simulink library "aerolibwindfilters"  (Simulink 6.0)
settings: Solver=ode45  SolverMode=SingleTasking  StartTime=0.0  StopTime=10.0  RelTol=1e-3
undefined symbols (not defined in the file or in its folder): dt, T_on
settings Model: Creator=sgage  LastModifiedBy=sgage  ExtModeAutoUpdateStatusClock=off
settings DataIOCC: SignalLoggingName=logsOut
settings OptimizationCC: BooleanDataType=off
settings DebuggingCC: CheckExecutionContextPreStartOutputMsg=on  CheckExecutionContextRuntimeOutputMsg=on  SolverPrmCheckMsg=none
settings HardwareCC: TargetUnknown=on
settings GRTTargetCC: LifeSpan=inf
settings SFSimCC: SFSimApplyToAllLibs=on  SFSimBuildMode=Incremental

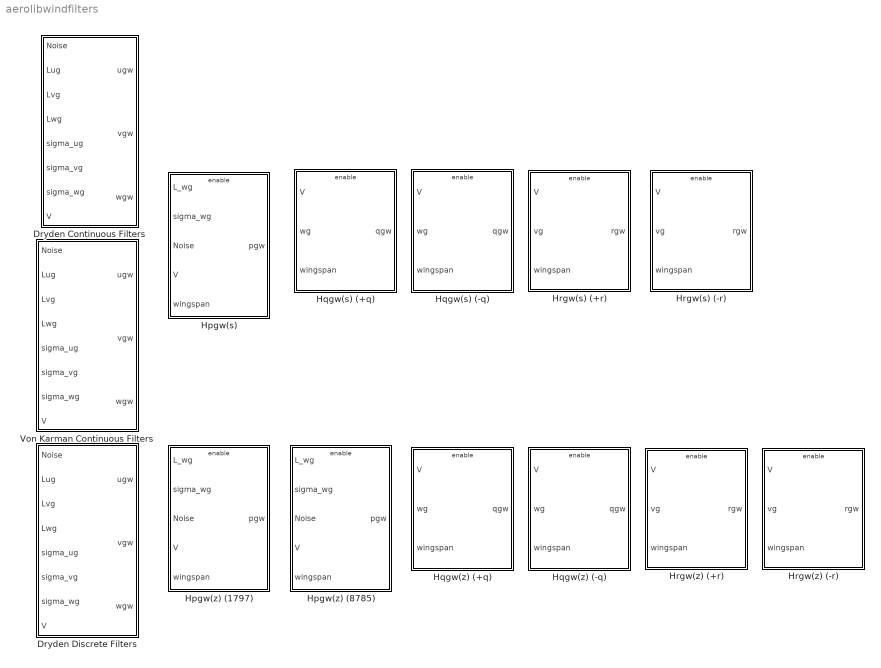
== system aerolibwindfilters ==
  Dryden Continuous Filters : Subsystem  PropExecContextAcrossSSBoundary=on
      mask Type: Dryden Continuous Filters
      mask Display: disp('Dryden\nCont.')
  Dryden Discrete Filters : Subsystem  PropExecContextAcrossSSBoundary=on
      mask Type: Dryden Discrete Filters
      mask Display: disp('Dryden\nDiscrete')
  Hpgw(s) : Subsystem  PropExecContextAcrossSSBoundary=on
      mask Type: Hpgw(s)
      mask Display: disp('P Cont.')
  Hpgw(z) (1797) : Subsystem  PropExecContextAcrossSSBoundary=on
      mask Type: Hpqw(z)
      mask Display: disp('P Disc.\n(1797)')
  Hpgw(z) (8785) : Subsystem  PropExecContextAcrossSSBoundary=on
      mask Type: Hpqw(z)
      mask Display: disp('P Disc.\n(8785)')
  Hqgw(s) (+q) : Subsystem  PropExecContextAcrossSSBoundary=on
      mask Type: Hqgw(s) (+q)
      mask Display: disp('+Q Cont.')
  Hqgw(s) (-q) : Subsystem  PropExecContextAcrossSSBoundary=on
      mask Type: Hqgw(s) (-q)
      mask Display: disp('-Q Cont.')
  Hqgw(z) (+q) : Subsystem  PropExecContextAcrossSSBoundary=on
      mask Type: Hqgw(z) (+q)
      mask Display: disp('+Q Disc.')
  Hqgw(z) (-q) : Subsystem  PropExecContextAcrossSSBoundary=on
      mask Type: Hqgw(z) (-q)
      mask Display: disp('-Q Disc.')
  Hrgw(s) (+r) : Subsystem  PropExecContextAcrossSSBoundary=on
      mask Type: Hrgw(s) (+r)
      mask Display: disp('+R Cont.')
  Hrgw(s) (-r) : Subsystem  PropExecContextAcrossSSBoundary=on
      mask Type: Hrgw(s) (-r)
      mask Display: disp('-R Cont.')
  Hrgw(z) (+r) : Subsystem  PropExecContextAcrossSSBoundary=on
      mask Type: Hrgw(z) (+r)
      mask Display: disp('+R Disc.')
  Hrgw(z) (-r) : Subsystem  PropExecContextAcrossSSBoundary=on
      mask Type: Hrgw(z) (-r)
      mask Display: disp('-R Disc.')
  Von Karman Continuous Filters : Subsystem  PropExecContextAcrossSSBoundary=on
      mask Type: Von Karman Continuous Filters
      mask Display: disp('VonKarman\nCont.')

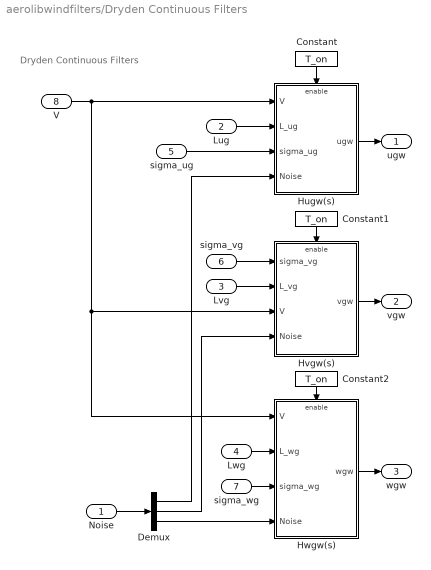
== system aerolibwindfilters/Dryden Continuous Filters ==
  note: Dryden Continuous Filters
  Noise : Inport  LatchInput=off
  Lug : Inport  Port=2  LatchInput=off
  Lvg : Inport  Port=3  LatchInput=off
  Lwg : Inport  Port=4  LatchInput=off
  sigma_ug : Inport  Port=5  LatchInput=off
  sigma_vg : Inport  Port=6  LatchInput=off
  sigma_wg : Inport  Port=7  LatchInput=off
  V : Inport  Port=8  LatchInput=off
  Constant : Constant  Orientation=down  Value=T_on
  Constant1 : Constant  Orientation=down  Value=T_on
  Constant2 : Constant  Orientation=down  Value=T_on
  Demux : Demux  Outputs=3
  Hugw(s) : Subsystem  PropExecContextAcrossSSBoundary=on
  Hvgw(s) : Subsystem  PropExecContextAcrossSSBoundary=on
  Hwgw(s) : Subsystem  PropExecContextAcrossSSBoundary=on
  ugw : Outport  OutputWhenDisabled=reset  InitialOutput=0
  vgw : Outport  Port=2  OutputWhenDisabled=reset  InitialOutput=0
  wgw : Outport  Port=3  OutputWhenDisabled=reset  InitialOutput=0
  wires:
  sigma_wg/1 -> Hwgw(s)/3(sigma_wg)
  Lwg/1 -> Hwgw(s)/2(L_wg)
  sigma_ug/1 -> Hugw(s)/3(sigma_ug)
  Lug/1 -> Hugw(s)/2(L_ug)
  V/1 -> Hwgw(s)/1(V), Hvgw(s)/3(V), Hugw(s)/1(V)
  Demux/3 -> Hwgw(s)/4(Noise)
  Hugw(s)/1(ugw) -> ugw/1
  Hvgw(s)/1(vgw) -> vgw/1
  Hwgw(s)/1(wgw) -> wgw/1
  Noise/1 -> Demux/1
  Demux/1 -> Hugw(s)/4(Noise)
  Demux/2 -> Hvgw(s)/4(Noise)
  Constant/1 -> Hugw(s)/Enable
  Constant1/1 -> Hvgw(s)/Enable
  Constant2/1 -> Hwgw(s)/Enable
  Lvg/1 -> Hvgw(s)/2(L_vg)
  sigma_vg/1 -> Hvgw(s)/1(sigma_vg)

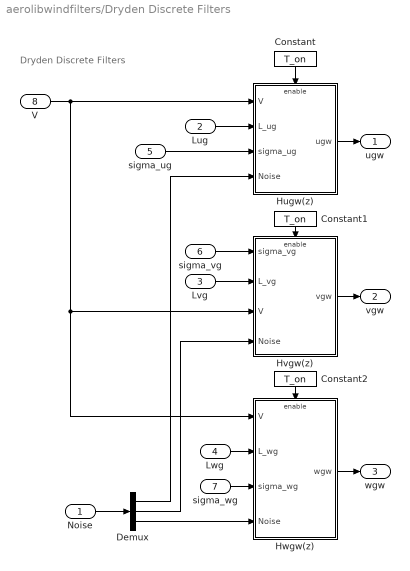
== system aerolibwindfilters/Dryden Discrete Filters ==
  note: Dryden Discrete Filters
  Noise : Inport  LatchInput=off
  Lug : Inport  Port=2  LatchInput=off
  Lvg : Inport  Port=3  LatchInput=off
  Lwg : Inport  Port=4  LatchInput=off
  sigma_ug : Inport  Port=5  LatchInput=off
  sigma_vg : Inport  Port=6  LatchInput=off
  sigma_wg : Inport  Port=7  LatchInput=off
  V : Inport  Port=8  LatchInput=off
  Constant : Constant  Orientation=down  Value=T_on
  Constant1 : Constant  Orientation=down  Value=T_on
  Constant2 : Constant  Orientation=down  Value=T_on
  Demux : Demux  Outputs=3
  Hugw(z) : Subsystem  PropExecContextAcrossSSBoundary=on
  Hvgw(z) : Subsystem  PropExecContextAcrossSSBoundary=on
  Hwgw(z) : Subsystem  PropExecContextAcrossSSBoundary=on
  ugw : Outport  InitialOutput=0
  vgw : Outport  Port=2  InitialOutput=0
  wgw : Outport  Port=3  InitialOutput=0
  wires:
  Lvg/1 -> Hvgw(z)/2(L_vg)
  Constant2/1 -> Hwgw(z)/Enable
  Constant1/1 -> Hvgw(z)/Enable
  Constant/1 -> Hugw(z)/Enable
  Demux/2 -> Hvgw(z)/4(Noise)
  Demux/1 -> Hugw(z)/4(Noise)
  Noise/1 -> Demux/1
  Hwgw(z)/1(wgw) -> wgw/1
  Hvgw(z)/1(vgw) -> vgw/1
  Hugw(z)/1(ugw) -> ugw/1
  Demux/3 -> Hwgw(z)/4(Noise)
  V/1 -> Hugw(z)/1(V), Hwgw(z)/1(V), Hvgw(z)/3(V)
  Lug/1 -> Hugw(z)/2(L_ug)
  sigma_ug/1 -> Hugw(z)/3(sigma_ug)
  Lwg/1 -> Hwgw(z)/2(L_wg)
  sigma_wg/1 -> Hwgw(z)/3(sigma_wg)
  sigma_vg/1 -> Hvgw(z)/1(sigma_vg)

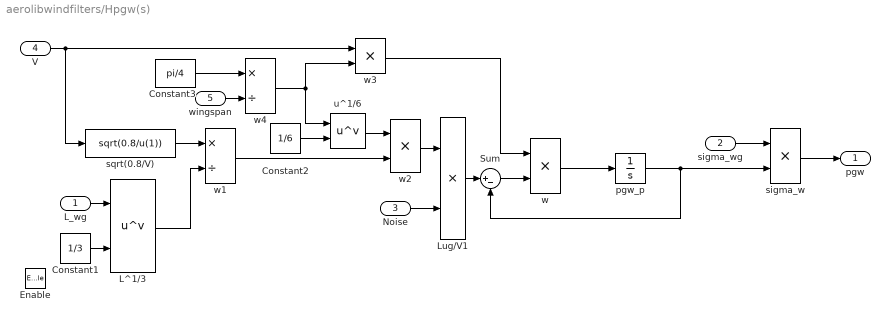
== system aerolibwindfilters/Hpgw(s) ==
  L_wg : Inport  LatchInput=off
  sigma_wg : Inport  Port=2  LatchInput=off
  Noise : Inport  Port=3  LatchInput=off
  V : Inport  Port=4  LatchInput=off
  wingspan : Inport  Port=5  LatchInput=off
  Enable : EnablePort  StatesWhenEnabling=reset
  Constant1 : Constant  Value=1/3
  Constant2 : Constant  Value=1/6
  Constant3 : Constant  Value=pi/4
  L^1/3 : Math  Operator=pow  SaturateOnIntegerOverflow=on
  Lug/V1 : Product  SaturateOnIntegerOverflow=on  InputSameDT=on
  Sum : Sum  Inputs=|+-  SaturateOnIntegerOverflow=on  InputSameDT=on
  pgw_p : Integrator
  sigma_w : Product  SaturateOnIntegerOverflow=on  InputSameDT=on
  sqrt(0.8/V) : Fcn  Expr=sqrt(0.8/u(1))
  u^1/6 : Math  Operator=pow  SaturateOnIntegerOverflow=on
  w : Product  SaturateOnIntegerOverflow=on  InputSameDT=on
  w1 : Product  Inputs=*/  SaturateOnIntegerOverflow=on  InputSameDT=on
  w2 : Product  SaturateOnIntegerOverflow=on  InputSameDT=on
  w3 : Product  SaturateOnIntegerOverflow=on  InputSameDT=on
  w4 : Product  Inputs=*/  SaturateOnIntegerOverflow=on  InputSameDT=on
  pgw : Outport  OutputWhenDisabled=reset  InitialOutput=0
  wires:
  wingspan/1 -> w4/2
  L^1/3/1 -> w1/2
  Noise/1 -> Lug/V1/2
  sqrt(0.8/V)/1 -> w1/1
  L_wg/1 -> L^1/3/1
  sigma_wg/1 -> sigma_w/1
  sigma_w/1 -> pgw/1
  w3/1 -> w/1
  Constant1/1 -> L^1/3/2
  pgw_p/1 -> Sum/2, sigma_w/2
  V/1 -> sqrt(0.8/V)/1, w3/1
  w/1 -> pgw_p/1
  Lug/V1/1 -> Sum/1
  Sum/1 -> w/2
  Constant2/1 -> u^1/6/2
  Constant3/1 -> w4/1
  w4/1 -> w3/2, u^1/6/1
  w2/1 -> Lug/V1/1
  u^1/6/1 -> w2/1
  w1/1 -> w2/2

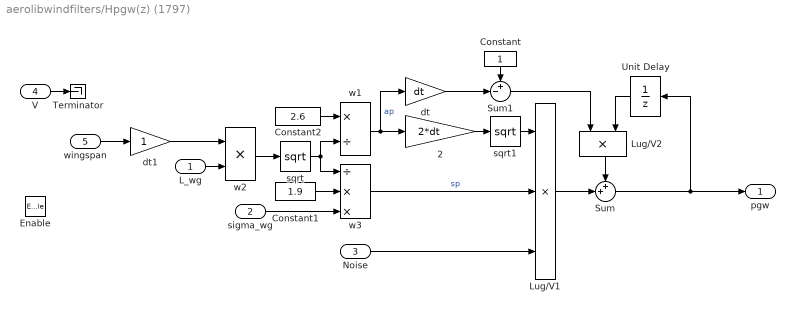
== system aerolibwindfilters/Hpgw(z) (1797) ==
  L_wg : Inport  LatchInput=off
  sigma_wg : Inport  Port=2  LatchInput=off
  Noise : Inport  Port=3  LatchInput=off
  V : Inport  Port=4  LatchInput=off
  wingspan : Inport  Port=5  LatchInput=off
  Enable : EnablePort  StatesWhenEnabling=reset
  2 : Gain  Gain=2*dt  SaturateOnIntegerOverflow=on
  Constant : Constant  Orientation=down
  Constant1 : Constant  Value=1.9
  Constant2 : Constant  Value=2.6
  Lug/V1 : Product  Inputs=3  SaturateOnIntegerOverflow=on  InputSameDT=on
  Lug/V2 : Product  Orientation=down  SaturateOnIntegerOverflow=on  InputSameDT=on
  Sum : Sum  Inputs=++|  SaturateOnIntegerOverflow=on  InputSameDT=on
  Sum1 : Sum  Inputs=+-|  SaturateOnIntegerOverflow=on  InputSameDT=on
  Terminator : Terminator
  Unit Delay : UnitDelay  Orientation=left  SampleTime=dt
  dt : Gain  Gain=dt  SaturateOnIntegerOverflow=on
  dt1 : Gain  SaturateOnIntegerOverflow=on
  sqrt : Math  Operator=sqrt  SaturateOnIntegerOverflow=on
  sqrt1 : Math  Operator=sqrt  SaturateOnIntegerOverflow=on
  w1 : Product  Inputs=*/  SaturateOnIntegerOverflow=on  InputSameDT=on
  w2 : Product  SaturateOnIntegerOverflow=on  InputSameDT=on
  w3 : Product  Inputs=/**  SaturateOnIntegerOverflow=on  InputSameDT=on
  pgw : Outport  OutputWhenDisabled=reset  InitialOutput=0
  wires:
  wingspan/1 -> dt1/1
  Lug/V2/1 -> Sum/1
  Unit Delay/1 -> Lug/V2/2
  Constant/1 -> Sum1/1
  Sum1/1 -> Lug/V2/1
  2/1 -> sqrt1/1
  dt/1 -> Sum1/2
  sqrt1/1 -> Lug/V1/1
  sigma_wg/1 -> w3/3
  w3/1 -> Lug/V1/2  "sp"
  Constant1/1 -> w3/2
  w1/1 -> 2/1, dt/1  "ap"
  Constant2/1 -> w1/1
  sqrt/1 -> w3/1, w1/2
  w2/1 -> sqrt/1
  L_wg/1 -> w2/2
  V/1 -> Terminator/1
  dt1/1 -> w2/1
  Lug/V1/1 -> Sum/2
  Sum/1 -> Unit Delay/1, pgw/1
  Noise/1 -> Lug/V1/3

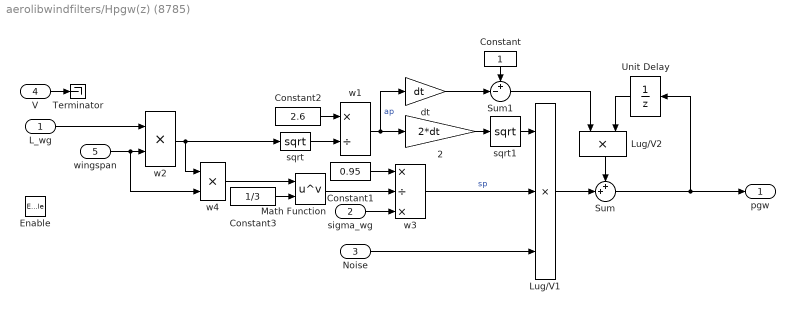
== system aerolibwindfilters/Hpgw(z) (8785) ==
  L_wg : Inport  LatchInput=off
  sigma_wg : Inport  Port=2  LatchInput=off
  Noise : Inport  Port=3  LatchInput=off
  V : Inport  Port=4  LatchInput=off
  wingspan : Inport  Port=5  LatchInput=off
  Enable : EnablePort  StatesWhenEnabling=reset
  2 : Gain  Gain=2*dt  SaturateOnIntegerOverflow=on
  Constant : Constant  Orientation=down
  Constant1 : Constant  Value=0.95
  Constant2 : Constant  Value=2.6
  Constant3 : Constant  Value=1/3
  Lug/V1 : Product  Inputs=3  SaturateOnIntegerOverflow=on  InputSameDT=on
  Lug/V2 : Product  Orientation=down  SaturateOnIntegerOverflow=on  InputSameDT=on
  Math Function : Math  Operator=pow  SaturateOnIntegerOverflow=on
  Sum : Sum  Inputs=++|  SaturateOnIntegerOverflow=on  InputSameDT=on
  Sum1 : Sum  Inputs=+-|  SaturateOnIntegerOverflow=on  InputSameDT=on
  Terminator : Terminator
  Unit Delay : UnitDelay  Orientation=left  SampleTime=dt
  dt : Gain  Gain=dt  SaturateOnIntegerOverflow=on
  sqrt : Math  Operator=sqrt  SaturateOnIntegerOverflow=on
  sqrt1 : Math  Operator=sqrt  SaturateOnIntegerOverflow=on
  w1 : Product  Inputs=*/  SaturateOnIntegerOverflow=on  InputSameDT=on
  w2 : Product  SaturateOnIntegerOverflow=on  InputSameDT=on
  w3 : Product  Inputs=*/*  SaturateOnIntegerOverflow=on  InputSameDT=on
  w4 : Product  SaturateOnIntegerOverflow=on  InputSameDT=on
  pgw : Outport  OutputWhenDisabled=reset  InitialOutput=0
  wires:
  Noise/1 -> Lug/V1/3
  Sum/1 -> pgw/1, Unit Delay/1
  Lug/V1/1 -> Sum/2
  V/1 -> Terminator/1
  wingspan/1 -> w2/2, w4/2
  w2/1 -> sqrt/1, w4/1
  sqrt/1 -> w1/2
  Constant2/1 -> w1/1
  w1/1 -> dt/1, 2/1  "ap"
  Constant1/1 -> w3/1
  w3/1 -> Lug/V1/2  "sp"
  sigma_wg/1 -> w3/3
  sqrt1/1 -> Lug/V1/1
  dt/1 -> Sum1/2
  2/1 -> sqrt1/1
  Sum1/1 -> Lug/V2/1
  Constant/1 -> Sum1/1
  Unit Delay/1 -> Lug/V2/2
  Lug/V2/1 -> Sum/1
  L_wg/1 -> w2/1
  Math Function/1 -> w3/2
  w4/1 -> Math Function/1
  Constant3/1 -> Math Function/2

== system aerolibwindfilters/Hqgw(s) (+q) ==
  V : Inport  LatchInput=off
  wg : Inport  Port=2  LatchInput=off
  wingspan : Inport  Port=3  LatchInput=off
  Enable : EnablePort  StatesWhenEnabling=reset
  Sum : Sum  Inputs=|+-  SaturateOnIntegerOverflow=on  InputSameDT=on
  pi/4 : Gain  Gain=pi/4  SaturateOnIntegerOverflow=on
  qgw_p : Integrator
  w : Product  Inputs=/**  SaturateOnIntegerOverflow=on  InputSameDT=on
  wg/V : Product  Inputs=/*  SaturateOnIntegerOverflow=on  InputSameDT=on
  qgw : Outport  OutputWhenDisabled=reset  InitialOutput=0
  wires:
  wingspan/1 -> w/1
  wg/1 -> wg/V/2
  wg/V/1 -> Sum/1
  Sum/1 -> w/3
  w/1 -> qgw/1, qgw_p/1
  V/1 -> wg/V/1, pi/4/1
  qgw_p/1 -> Sum/2
  pi/4/1 -> w/2

== system aerolibwindfilters/Hqgw(s) (-q) ==
  V : Inport  LatchInput=off
  wg : Inport  Port=2  LatchInput=off
  wingspan : Inport  Port=3  LatchInput=off
  Enable : EnablePort  StatesWhenEnabling=reset
  -1 : Gain  Gain=-1  SaturateOnIntegerOverflow=on
  Sum : Sum  Inputs=|+-  SaturateOnIntegerOverflow=on  InputSameDT=on
  pi/4 : Gain  Gain=pi/4  SaturateOnIntegerOverflow=on
  qgw_p : Integrator
  w : Product  Inputs=/**  SaturateOnIntegerOverflow=on  InputSameDT=on
  wg/V : Product  Inputs=/*  SaturateOnIntegerOverflow=on  InputSameDT=on
  qgw : Outport  OutputWhenDisabled=reset  InitialOutput=0
  wires:
  pi/4/1 -> w/2
  qgw_p/1 -> Sum/2
  V/1 -> pi/4/1, wg/V/1
  w/1 -> -1/1, qgw_p/1
  Sum/1 -> w/3
  wg/V/1 -> Sum/1
  wg/1 -> wg/V/2
  wingspan/1 -> w/1
  -1/1 -> qgw/1

== system aerolibwindfilters/Hqgw(z) (+q) ==
  V : Inport  LatchInput=off
  wg : Inport  Port=2  LatchInput=off
  wingspan : Inport  Port=3  LatchInput=off
  Enable : EnablePort  StatesWhenEnabling=reset
  Constant : Constant  Orientation=down
  Lug/V2 : Product  Orientation=down  SaturateOnIntegerOverflow=on  InputSameDT=on
  Sum1 : Sum  Inputs=++|  SaturateOnIntegerOverflow=on  InputSameDT=on
  Sum2 : Sum  Inputs=+-|  SaturateOnIntegerOverflow=on  InputSameDT=on
  Sum3 : Sum  Inputs=|+-  SaturateOnIntegerOverflow=on  InputSameDT=on
  Unit Delay : UnitDelay  Orientation=left  SampleTime=dt
  Unit Delay1 : UnitDelay  SampleTime=dt
  dt : Gain  Gain=dt  SaturateOnIntegerOverflow=on
  dt1 : Gain  Gain=4/pi  SaturateOnIntegerOverflow=on
  w1 : Product  Inputs=*/  SaturateOnIntegerOverflow=on  InputSameDT=on
  w2 : Product  Inputs=/*  SaturateOnIntegerOverflow=on  InputSameDT=on
  qgw : Outport  OutputWhenDisabled=reset  InitialOutput=0
  wires:
  wingspan/1 -> dt1/1
  wg/1 -> Unit Delay1/1, Sum3/1
  Unit Delay1/1 -> Sum3/2
  Sum3/1 -> w2/2
  w1/1 -> dt/1  "aq"
  Lug/V2/1 -> Sum1/1
  Unit Delay/1 -> Lug/V2/2
  Constant/1 -> Sum2/1
  Sum2/1 -> Lug/V2/1
  dt/1 -> Sum2/2
  w2/1 -> Sum1/2
  Sum1/1 -> qgw/1, Unit Delay/1
  dt1/1 -> w2/1, w1/2
  V/1 -> w1/1

== system aerolibwindfilters/Hqgw(z) (-q) ==
  V : Inport  LatchInput=off
  wg : Inport  Port=2  LatchInput=off
  wingspan : Inport  Port=3  LatchInput=off
  Enable : EnablePort  StatesWhenEnabling=reset
  Constant : Constant  Orientation=down
  Lug/V2 : Product  Orientation=down  SaturateOnIntegerOverflow=on  InputSameDT=on
  Sum1 : Sum  Inputs=+-|  SaturateOnIntegerOverflow=on  InputSameDT=on
  Sum2 : Sum  Inputs=+-|  SaturateOnIntegerOverflow=on  InputSameDT=on
  Sum3 : Sum  Inputs=|+-  SaturateOnIntegerOverflow=on  InputSameDT=on
  Unit Delay : UnitDelay  Orientation=left  SampleTime=dt
  Unit Delay1 : UnitDelay  SampleTime=dt
  dt : Gain  Gain=dt  SaturateOnIntegerOverflow=on
  dt1 : Gain  Gain=4/pi  SaturateOnIntegerOverflow=on
  w1 : Product  Inputs=*/  SaturateOnIntegerOverflow=on  InputSameDT=on
  w2 : Product  Inputs=/*  SaturateOnIntegerOverflow=on  InputSameDT=on
  qgw : Outport  OutputWhenDisabled=reset  InitialOutput=0
  wires:
  V/1 -> w1/1
  dt1/1 -> w1/2, w2/1
  Sum1/1 -> Unit Delay/1, qgw/1
  w2/1 -> Sum1/2
  dt/1 -> Sum2/2
  Sum2/1 -> Lug/V2/1
  Constant/1 -> Sum2/1
  Unit Delay/1 -> Lug/V2/2
  Lug/V2/1 -> Sum1/1
  w1/1 -> dt/1  "aq"
  Sum3/1 -> w2/2
  Unit Delay1/1 -> Sum3/2
  wg/1 -> Sum3/1, Unit Delay1/1
  wingspan/1 -> dt1/1

== system aerolibwindfilters/Hrgw(s) (+r) ==
  V : Inport  LatchInput=off
  vg : Inport  Port=2  LatchInput=off
  wingspan : Inport  Port=3  LatchInput=off
  Enable : EnablePort  StatesWhenEnabling=reset
  Sum : Sum  Inputs=|+-  SaturateOnIntegerOverflow=on  InputSameDT=on
  pi/3 : Gain  Gain=pi/3  SaturateOnIntegerOverflow=on
  rgw_p : Integrator
  vg/V : Product  Inputs=/*  SaturateOnIntegerOverflow=on  InputSameDT=on
  w : Product  Inputs=/**  SaturateOnIntegerOverflow=on  InputSameDT=on
  rgw : Outport  OutputWhenDisabled=reset  InitialOutput=0
  wires:
  wingspan/1 -> w/1
  vg/V/1 -> Sum/1
  vg/1 -> vg/V/2
  pi/3/1 -> w/2
  V/1 -> vg/V/1, pi/3/1
  w/1 -> rgw/1, rgw_p/1
  Sum/1 -> w/3
  rgw_p/1 -> Sum/2

== system aerolibwindfilters/Hrgw(s) (-r) ==
  V : Inport  LatchInput=off
  vg : Inport  Port=2  LatchInput=off
  wingspan : Inport  Port=3  LatchInput=off
  Enable : EnablePort  StatesWhenEnabling=reset
  -1 : Gain  Gain=-1  SaturateOnIntegerOverflow=on
  Sum : Sum  Inputs=|+-  SaturateOnIntegerOverflow=on  InputSameDT=on
  pi/3 : Gain  Gain=pi/3  SaturateOnIntegerOverflow=on
  rgw_p : Integrator
  vg/V : Product  Inputs=/*  SaturateOnIntegerOverflow=on  InputSameDT=on
  w : Product  Inputs=/**  SaturateOnIntegerOverflow=on  InputSameDT=on
  rgw : Outport  OutputWhenDisabled=reset  InitialOutput=0
  wires:
  Sum/1 -> w/3
  w/1 -> -1/1, rgw_p/1
  V/1 -> pi/3/1, vg/V/1
  rgw_p/1 -> Sum/2
  pi/3/1 -> w/2
  vg/1 -> vg/V/2
  vg/V/1 -> Sum/1
  -1/1 -> rgw/1
  wingspan/1 -> w/1

== system aerolibwindfilters/Hrgw(z) (+r) ==
  V : Inport  LatchInput=off
  vg : Inport  Port=2  LatchInput=off
  wingspan : Inport  Port=3  LatchInput=off
  Enable : EnablePort  StatesWhenEnabling=reset
  Constant : Constant  Orientation=down
  Lug/V2 : Product  Orientation=down  SaturateOnIntegerOverflow=on  InputSameDT=on
  Sum1 : Sum  Inputs=++|  SaturateOnIntegerOverflow=on  InputSameDT=on
  Sum2 : Sum  Inputs=+-|  SaturateOnIntegerOverflow=on  InputSameDT=on
  Sum3 : Sum  Inputs=|+-  SaturateOnIntegerOverflow=on  InputSameDT=on
  Unit Delay : UnitDelay  Orientation=left  SampleTime=dt
  Unit Delay1 : UnitDelay  SampleTime=dt
  dt : Gain  Gain=dt  SaturateOnIntegerOverflow=on
  dt1 : Gain  Gain=3/pi  SaturateOnIntegerOverflow=on
  w1 : Product  Inputs=*/  SaturateOnIntegerOverflow=on  InputSameDT=on
  w2 : Product  Inputs=/*  SaturateOnIntegerOverflow=on  InputSameDT=on
  rgw : Outport  OutputWhenDisabled=reset  InitialOutput=0
  wires:
  wingspan/1 -> dt1/1
  Unit Delay1/1 -> Sum3/2
  vg/1 -> Sum3/1, Unit Delay1/1
  Sum3/1 -> w2/2
  w1/1 -> dt/1  "ar"
  Lug/V2/1 -> Sum1/1
  Unit Delay/1 -> Lug/V2/2
  Constant/1 -> Sum2/1
  Sum2/1 -> Lug/V2/1
  dt/1 -> Sum2/2
  w2/1 -> Sum1/2
  Sum1/1 -> rgw/1, Unit Delay/1
  dt1/1 -> w1/2, w2/1
  V/1 -> w1/1

== system aerolibwindfilters/Hrgw(z) (-r) ==
  V : Inport  LatchInput=off
  vg : Inport  Port=2  LatchInput=off
  wingspan : Inport  Port=3  LatchInput=off
  Enable : EnablePort  StatesWhenEnabling=reset
  Constant : Constant  Orientation=down
  Lug/V2 : Product  Orientation=down  SaturateOnIntegerOverflow=on  InputSameDT=on
  Sum1 : Sum  Inputs=+-|  SaturateOnIntegerOverflow=on  InputSameDT=on
  Sum2 : Sum  Inputs=+-|  SaturateOnIntegerOverflow=on  InputSameDT=on
  Sum3 : Sum  Inputs=|+-  SaturateOnIntegerOverflow=on  InputSameDT=on
  Unit Delay : UnitDelay  Orientation=left  SampleTime=dt
  Unit Delay1 : UnitDelay  SampleTime=dt
  dt : Gain  Gain=dt  SaturateOnIntegerOverflow=on
  dt1 : Gain  Gain=3/pi  SaturateOnIntegerOverflow=on
  w1 : Product  Inputs=*/  SaturateOnIntegerOverflow=on  InputSameDT=on
  w2 : Product  Inputs=/*  SaturateOnIntegerOverflow=on  InputSameDT=on
  rgw : Outport  OutputWhenDisabled=reset  InitialOutput=0
  wires:
  wingspan/1 -> dt1/1
  V/1 -> w1/1
  dt1/1 -> w2/1, w1/2
  Sum1/1 -> Unit Delay/1, rgw/1
  w2/1 -> Sum1/2
  dt/1 -> Sum2/2
  Sum2/1 -> Lug/V2/1
  Constant/1 -> Sum2/1
  Unit Delay/1 -> Lug/V2/2
  Lug/V2/1 -> Sum1/1
  w1/1 -> dt/1  "ar"
  Sum3/1 -> w2/2
  vg/1 -> Unit Delay1/1, Sum3/1
  Unit Delay1/1 -> Sum3/2

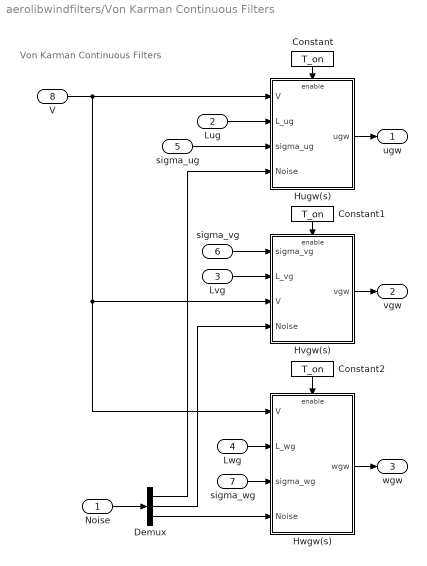
== system aerolibwindfilters/Von Karman Continuous Filters ==
  note: Von Karman Continuous Filters
  Noise : Inport  LatchInput=off
  Lug : Inport  Port=2  LatchInput=off
  Lvg : Inport  Port=3  LatchInput=off
  Lwg : Inport  Port=4  LatchInput=off
  sigma_ug : Inport  Port=5  LatchInput=off
  sigma_vg : Inport  Port=6  LatchInput=off
  sigma_wg : Inport  Port=7  LatchInput=off
  V : Inport  Port=8  LatchInput=off
  Constant : Constant  Orientation=down  Value=T_on
  Constant1 : Constant  Orientation=down  Value=T_on
  Constant2 : Constant  Orientation=down  Value=T_on
  Demux : Demux  Outputs=3
  Hugw(s) : Subsystem  PropExecContextAcrossSSBoundary=on
  Hvgw(s) : Subsystem  PropExecContextAcrossSSBoundary=on
  Hwgw(s) : Subsystem  PropExecContextAcrossSSBoundary=on
  ugw : Outport  OutputWhenDisabled=reset  InitialOutput=0
  vgw : Outport  Port=2  OutputWhenDisabled=reset  InitialOutput=0
  wgw : Outport  Port=3  OutputWhenDisabled=reset  InitialOutput=0
  wires:
  sigma_wg/1 -> Hwgw(s)/3(sigma_wg)
  Lwg/1 -> Hwgw(s)/2(L_wg)
  sigma_ug/1 -> Hugw(s)/3(sigma_ug)
  Lug/1 -> Hugw(s)/2(L_ug)
  V/1 -> Hwgw(s)/1(V), Hvgw(s)/3(V), Hugw(s)/1(V)
  Demux/3 -> Hwgw(s)/4(Noise)
  Hugw(s)/1(ugw) -> ugw/1
  Hvgw(s)/1(vgw) -> vgw/1
  Hwgw(s)/1(wgw) -> wgw/1
  Noise/1 -> Demux/1
  Demux/1 -> Hugw(s)/4(Noise)
  Demux/2 -> Hvgw(s)/4(Noise)
  Constant/1 -> Hugw(s)/Enable
  Constant2/1 -> Hwgw(s)/Enable
  Constant1/1 -> Hvgw(s)/Enable
  Lvg/1 -> Hvgw(s)/2(L_vg)
  sigma_vg/1 -> Hvgw(s)/1(sigma_vg)

== system aerolibwindfilters/Dryden Continuous Filters/Hugw(s) ==
  V : Inport  LatchInput=off
  L_ug : Inport  Port=2  LatchInput=off
  sigma_ug : Inport  Port=3  LatchInput=off
  Noise : Inport  Port=4  LatchInput=off
  Enable : EnablePort  StatesWhenEnabling=reset
  (2/pi) : Gain  Gain=2/pi  SaturateOnIntegerOverflow=on
  Lug/V : Product  Inputs=*/  SaturateOnIntegerOverflow=on  InputSameDT=on
  Lug/V1 : Product  SaturateOnIntegerOverflow=on  InputSameDT=on
  Math Function : Math  Operator=sqrt  SaturateOnIntegerOverflow=on
  Sum : Sum  Inputs=|+-  SaturateOnIntegerOverflow=on  InputSameDT=on
  ug_p : Integrator
  w : Product  Inputs=/*  SaturateOnIntegerOverflow=on  InputSameDT=on
  w1 : Product  SaturateOnIntegerOverflow=on  InputSameDT=on
  ugw : Outport  OutputWhenDisabled=reset  InitialOutput=0
  wires:
  Lug/V/1 -> w/1, (2/pi)/1
  Sum/1 -> w/2
  Lug/V1/1 -> Sum/1
  w/1 -> ug_p/1
  V/1 -> Lug/V/2
  L_ug/1 -> Lug/V/1
  ug_p/1 -> Sum/2, w1/2
  w1/1 -> ugw/1
  sigma_ug/1 -> w1/1
  Noise/1 -> Lug/V1/2
  (2/pi)/1 -> Math Function/1
  Math Function/1 -> Lug/V1/1

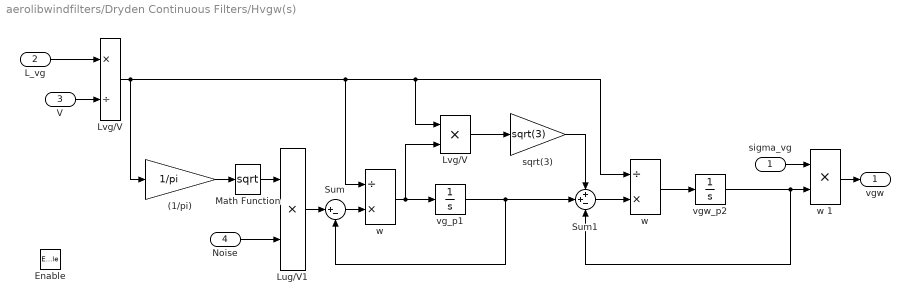
== system aerolibwindfilters/Dryden Continuous Filters/Hvgw(s) ==
  sigma_vg : Inport  LatchInput=off
  L_vg : Inport  Port=2  LatchInput=off
  V : Inport  Port=3  LatchInput=off
  Noise : Inport  Port=4  LatchInput=off
  Enable : EnablePort  StatesWhenEnabling=reset
  (1/pi) : Gain  Gain=1/pi  SaturateOnIntegerOverflow=on
  Lug/V1 : Product  SaturateOnIntegerOverflow=on  InputSameDT=on
  Lvg/V : Product  Inputs=*/  SaturateOnIntegerOverflow=on  InputSameDT=on
  "Lvg/V " : Product  SaturateOnIntegerOverflow=on  InputSameDT=on
  Math Function : Math  Operator=sqrt  SaturateOnIntegerOverflow=on
  Sum : Sum  Inputs=|+-  SaturateOnIntegerOverflow=on  InputSameDT=on
  Sum1 : Sum  Inputs=++-  SaturateOnIntegerOverflow=on  InputSameDT=on
  sqrt(3) : Gain  Gain=sqrt(3)  SaturateOnIntegerOverflow=on
  vg_p1 : Integrator
  vgw_p2 : Integrator
  w : Product  Inputs=/*  SaturateOnIntegerOverflow=on  InputSameDT=on
  "w " : Product  Inputs=/*  SaturateOnIntegerOverflow=on  InputSameDT=on
  w 1 : Product  SaturateOnIntegerOverflow=on  InputSameDT=on
  vgw : Outport  OutputWhenDisabled=reset  InitialOutput=0
  wires:
  (1/pi)/1 -> Math Function/1
  sqrt(3)/1 -> Sum1/1
  "Lvg/V "/1 -> sqrt(3)/1
  "w "/1 -> vgw_p2/1
  Sum1/1 -> "w "/2
  vgw_p2/1 -> Sum1/3, w 1/2
  vg_p1/1 -> Sum1/2, Sum/2
  L_vg/1 -> Lvg/V/1
  V/1 -> Lvg/V/2
  w/1 -> "Lvg/V "/2, vg_p1/1
  Lug/V1/1 -> Sum/1
  Sum/1 -> w/2
  Lvg/V/1 -> "Lvg/V "/1, "w "/1, w/1, (1/pi)/1
  sigma_vg/1 -> w 1/1
  Noise/1 -> Lug/V1/2
  w 1/1 -> vgw/1
  Math Function/1 -> Lug/V1/1

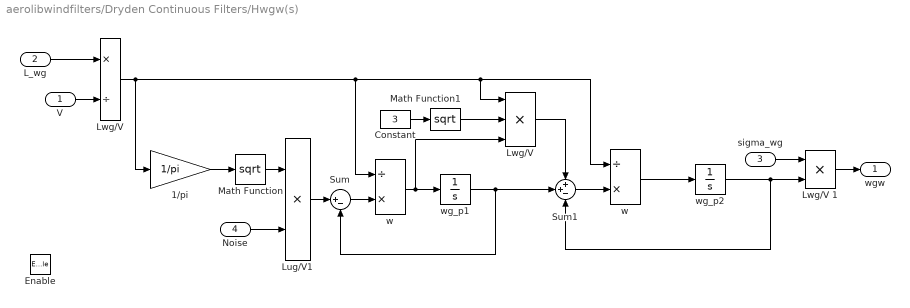
== system aerolibwindfilters/Dryden Continuous Filters/Hwgw(s) ==
  V : Inport  LatchInput=off
  L_wg : Inport  Port=2  LatchInput=off
  sigma_wg : Inport  Port=3  LatchInput=off
  Noise : Inport  Port=4  LatchInput=off
  Enable : EnablePort  StatesWhenEnabling=reset
  1/pi : Gain  Gain=1/pi  SaturateOnIntegerOverflow=on
  Constant : Constant  Value=3
  Lug/V1 : Product  SaturateOnIntegerOverflow=on  InputSameDT=on
  Lwg/V : Product  Inputs=*/  SaturateOnIntegerOverflow=on  InputSameDT=on
  "Lwg/V " : Product  Inputs=3  SaturateOnIntegerOverflow=on  InputSameDT=on
  Lwg/V 1 : Product  SaturateOnIntegerOverflow=on  InputSameDT=on
  Math Function : Math  Operator=sqrt  SaturateOnIntegerOverflow=on
  Math Function1 : Math  Operator=sqrt  SaturateOnIntegerOverflow=on
  Sum : Sum  Inputs=|+-  SaturateOnIntegerOverflow=on  InputSameDT=on
  Sum1 : Sum  Inputs=++-  SaturateOnIntegerOverflow=on  InputSameDT=on
  w : Product  Inputs=/*  SaturateOnIntegerOverflow=on  InputSameDT=on
  "w " : Product  Inputs=/*  SaturateOnIntegerOverflow=on  InputSameDT=on
  wg_p1 : Integrator
  wg_p2 : Integrator
  wgw : Outport  OutputWhenDisabled=reset  InitialOutput=0
  wires:
  Math Function/1 -> Lug/V1/1
  Lwg/V/1 -> w/1, "w "/1, "Lwg/V "/1, 1/pi/1
  Sum/1 -> w/2
  Lug/V1/1 -> Sum/1
  w/1 -> "Lwg/V "/3, wg_p1/1
  V/1 -> Lwg/V/2
  L_wg/1 -> Lwg/V/1
  wg_p1/1 -> Sum/2, Sum1/2
  wg_p2/1 -> Sum1/3, Lwg/V 1/2
  Sum1/1 -> "w "/2
  "w "/1 -> wg_p2/1
  "Lwg/V "/1 -> Sum1/1
  Lwg/V 1/1 -> wgw/1
  sigma_wg/1 -> Lwg/V 1/1
  Noise/1 -> Lug/V1/2
  1/pi/1 -> Math Function/1
  Math Function1/1 -> "Lwg/V "/2
  Constant/1 -> Math Function1/1

== system aerolibwindfilters/Dryden Discrete Filters/Hugw(z) ==
  V : Inport  LatchInput=off
  L_ug : Inport  Port=2  LatchInput=off
  sigma_ug : Inport  Port=3  LatchInput=off
  Noise : Inport  Port=4  LatchInput=off
  Enable : EnablePort  StatesWhenEnabling=reset
  2 : Gain  Gain=2*dt  SaturateOnIntegerOverflow=on
  Constant : Constant  Orientation=down
  Lug/V1 : Product  Inputs=3  SaturateOnIntegerOverflow=on  InputSameDT=on
  Lug/V2 : Product  Orientation=down  SaturateOnIntegerOverflow=on  InputSameDT=on
  Math Function : Math  Operator=sqrt  SaturateOnIntegerOverflow=on
  Sum : Sum  Inputs=++|  SaturateOnIntegerOverflow=on  InputSameDT=on
  Sum1 : Sum  Inputs=+-|  SaturateOnIntegerOverflow=on  InputSameDT=on
  Unit Delay : UnitDelay  Orientation=left  SampleTime=dt
  V/Lug : Product  Inputs=/*  SaturateOnIntegerOverflow=on  InputSameDT=on
  dt : Gain  Gain=dt  SaturateOnIntegerOverflow=on
  ugw : Outport  OutputWhenDisabled=reset  InitialOutput=0
  wires:
  Math Function/1 -> Lug/V1/1
  2/1 -> Math Function/1
  Noise/1 -> Lug/V1/2
  Sum/1 -> ugw/1, Unit Delay/1
  L_ug/1 -> V/Lug/1
  V/1 -> V/Lug/2
  Lug/V1/1 -> Sum/2
  V/Lug/1 -> 2/1, dt/1
  sigma_ug/1 -> Lug/V1/3
  dt/1 -> Sum1/2
  Lug/V2/1 -> Sum/1
  Sum1/1 -> Lug/V2/1
  Unit Delay/1 -> Lug/V2/2
  Constant/1 -> Sum1/1

== system aerolibwindfilters/Dryden Discrete Filters/Hvgw(z) ==
  sigma_vg : Inport  LatchInput=off
  L_vg : Inport  Port=2  LatchInput=off
  V : Inport  Port=3  LatchInput=off
  Noise : Inport  Port=4  LatchInput=off
  Enable : EnablePort  StatesWhenEnabling=reset
  2 : Gain  Gain=2*dt  SaturateOnIntegerOverflow=on
  Constant : Constant  Orientation=down
  Lug/V1 : Product  Inputs=3  SaturateOnIntegerOverflow=on  InputSameDT=on
  Lug/V2 : Product  Orientation=down  SaturateOnIntegerOverflow=on  InputSameDT=on
  Math Function : Math  Operator=sqrt  SaturateOnIntegerOverflow=on
  Sum : Sum  Inputs=++|  SaturateOnIntegerOverflow=on  InputSameDT=on
  Sum1 : Sum  Inputs=+-|  SaturateOnIntegerOverflow=on  InputSameDT=on
  Unit Delay : UnitDelay  Orientation=left  SampleTime=dt
  V/Lvg : Product  Inputs=/*  SaturateOnIntegerOverflow=on  InputSameDT=on
  dt : Gain  Gain=dt  SaturateOnIntegerOverflow=on
  vgw : Outport  OutputWhenDisabled=reset  InitialOutput=0
  wires:
  Math Function/1 -> Lug/V1/1
  2/1 -> Math Function/1
  Noise/1 -> Lug/V1/2
  Sum/1 -> Unit Delay/1, vgw/1
  L_vg/1 -> V/Lvg/1
  V/1 -> V/Lvg/2
  Lug/V1/1 -> Sum/2
  V/Lvg/1 -> dt/1, 2/1
  sigma_vg/1 -> Lug/V1/3
  dt/1 -> Sum1/2
  Lug/V2/1 -> Sum/1
  Sum1/1 -> Lug/V2/1
  Unit Delay/1 -> Lug/V2/2
  Constant/1 -> Sum1/1

== system aerolibwindfilters/Dryden Discrete Filters/Hwgw(z) ==
  V : Inport  LatchInput=off
  L_wg : Inport  Port=2  LatchInput=off
  sigma_wg : Inport  Port=3  LatchInput=off
  Noise : Inport  Port=4  LatchInput=off
  Enable : EnablePort  StatesWhenEnabling=reset
  2 : Gain  Gain=2*dt  SaturateOnIntegerOverflow=on
  Constant : Constant  Orientation=down
  Lug/V1 : Product  Inputs=3  SaturateOnIntegerOverflow=on  InputSameDT=on
  Lug/V2 : Product  Orientation=down  SaturateOnIntegerOverflow=on  InputSameDT=on
  Math Function : Math  Operator=sqrt  SaturateOnIntegerOverflow=on
  Sum : Sum  Inputs=++|  SaturateOnIntegerOverflow=on  InputSameDT=on
  Sum1 : Sum  Inputs=+-|  SaturateOnIntegerOverflow=on  InputSameDT=on
  Unit Delay : UnitDelay  Orientation=left  SampleTime=dt
  V/Lwg : Product  Inputs=/*  SaturateOnIntegerOverflow=on  InputSameDT=on
  dt : Gain  Gain=dt  SaturateOnIntegerOverflow=on
  wgw : Outport  OutputWhenDisabled=reset  InitialOutput=0
  wires:
  Math Function/1 -> Lug/V1/1
  2/1 -> Math Function/1
  Noise/1 -> Lug/V1/2
  Sum/1 -> wgw/1, Unit Delay/1
  L_wg/1 -> V/Lwg/1
  V/1 -> V/Lwg/2
  Lug/V1/1 -> Sum/2
  V/Lwg/1 -> 2/1, dt/1
  sigma_wg/1 -> Lug/V1/3
  dt/1 -> Sum1/2
  Lug/V2/1 -> Sum/1
  Sum1/1 -> Lug/V2/1
  Unit Delay/1 -> Lug/V2/2
  Constant/1 -> Sum1/1

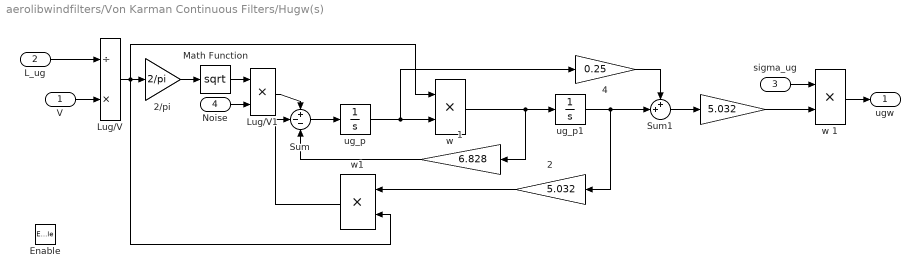
== system aerolibwindfilters/Von Karman Continuous Filters/Hugw(s) ==
  V : Inport  LatchInput=off
  L_ug : Inport  Port=2  LatchInput=off
  sigma_ug : Inport  Port=3  LatchInput=off
  Noise : Inport  Port=4  LatchInput=off
  Enable : EnablePort  StatesWhenEnabling=reset
  " " : Gain  Gain=5.032  SaturateOnIntegerOverflow=on
  " 1" : Gain  Orientation=left  Gain=6.828  SaturateOnIntegerOverflow=on
  " 2" : Gain  Orientation=left  Gain=5.032  SaturateOnIntegerOverflow=on
  2/pi : Gain  Gain=2/pi  SaturateOnIntegerOverflow=on
  4 : Gain  Gain=0.25  SaturateOnIntegerOverflow=on
  Lug/V : Product  Inputs=/*  SaturateOnIntegerOverflow=on  InputSameDT=on
  Lug/V1 : Product  SaturateOnIntegerOverflow=on  InputSameDT=on
  Math Function : Math  Operator=sqrt  SaturateOnIntegerOverflow=on
  Sum : Sum  Inputs=+--  SaturateOnIntegerOverflow=on  InputSameDT=on
  Sum1 : Sum  Inputs=++|  SaturateOnIntegerOverflow=on  InputSameDT=on
  ug_p : Integrator
  ug_p1 : Integrator
  w : Product  SaturateOnIntegerOverflow=on  InputSameDT=on
  w 1 : Product  SaturateOnIntegerOverflow=on  InputSameDT=on
  w1 : Product  Orientation=left  SaturateOnIntegerOverflow=on  InputSameDT=on
  ugw : Outport  OutputWhenDisabled=reset  InitialOutput=0
  wires:
  Math Function/1 -> Lug/V1/1
  Noise/1 -> Lug/V1/2
  ug_p1/1 -> Sum1/2, " 2"/1
  L_ug/1 -> Lug/V/1
  V/1 -> Lug/V/2
  Sum/1 -> ug_p/1
  Lug/V/1 -> w/1, w1/2, 2/pi/1
  Lug/V1/1 -> Sum/1
  w/1 -> " 1"/1, ug_p1/1
  ug_p/1 -> w/2, 4/1
  4/1 -> Sum1/1
  Sum1/1 -> " "/1
  w1/1 -> Sum/2
  " 1"/1 -> Sum/3
  sigma_ug/1 -> w 1/1
  w 1/1 -> ugw/1
  " 2"/1 -> w1/1
  " "/1 -> w 1/2
  2/pi/1 -> Math Function/1

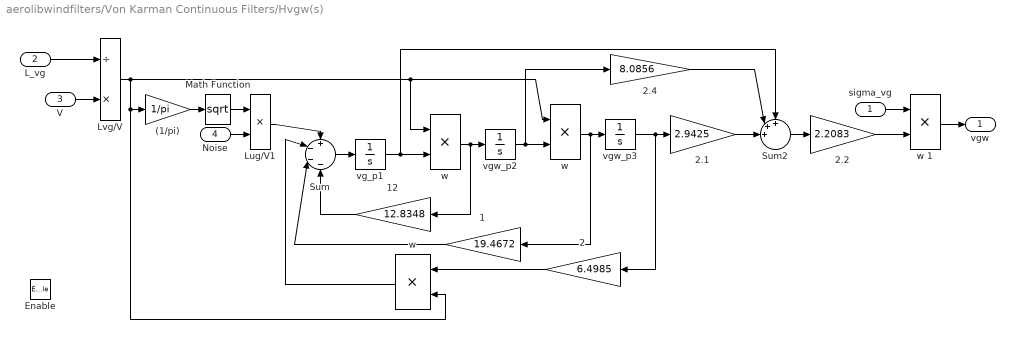
== system aerolibwindfilters/Von Karman Continuous Filters/Hvgw(s) ==
  sigma_vg : Inport  LatchInput=off
  L_vg : Inport  Port=2  LatchInput=off
  V : Inport  Port=3  LatchInput=off
  Noise : Inport  Port=4  LatchInput=off
  Enable : EnablePort  StatesWhenEnabling=reset
  " w" : Product  Orientation=left  SaturateOnIntegerOverflow=on  InputSameDT=on
  (1/pi) : Gain  Gain=1/pi  SaturateOnIntegerOverflow=on
  1 : Gain  Orientation=left  Gain=19.4672  SaturateOnIntegerOverflow=on
  12 : Gain  Orientation=left  Gain=12.8348  SaturateOnIntegerOverflow=on
  2 : Gain  Orientation=left  Gain=6.4985  SaturateOnIntegerOverflow=on
  2.1 : Gain  Gain=2.9425  SaturateOnIntegerOverflow=on
  2.2 : Gain  Gain=2.2083  SaturateOnIntegerOverflow=on
  2.4 : Gain  Gain=8.0856  SaturateOnIntegerOverflow=on
  Lug/V1 : Product  SaturateOnIntegerOverflow=on  InputSameDT=on
  Lvg/V : Product  Inputs=/*  SaturateOnIntegerOverflow=on  InputSameDT=on
  Math Function : Math  Operator=sqrt  SaturateOnIntegerOverflow=on
  Sum : Sum  Inputs=+---  SaturateOnIntegerOverflow=on  InputSameDT=on
  Sum2 : Sum  Inputs=+++||  SaturateOnIntegerOverflow=on  InputSameDT=on
  vg_p1 : Integrator
  vgw_p2 : Integrator
  vgw_p3 : Integrator
  w : Product  SaturateOnIntegerOverflow=on  InputSameDT=on
  "w " : Product  SaturateOnIntegerOverflow=on  InputSameDT=on
  w 1 : Product  SaturateOnIntegerOverflow=on  InputSameDT=on
  vgw : Outport  OutputWhenDisabled=reset  InitialOutput=0
  wires:
  Math Function/1 -> Lug/V1/1
  Noise/1 -> Lug/V1/2
  sigma_vg/1 -> w 1/1
  Lvg/V/1 -> "w "/1, w/1, (1/pi)/1, " w"/2
  Sum/1 -> vg_p1/1
  Lug/V1/1 -> Sum/1
  V/1 -> Lvg/V/2
  L_vg/1 -> Lvg/V/1
  vg_p1/1 -> "w "/2, Sum2/1
  "w "/1 -> 12/1, vgw_p2/1
  (1/pi)/1 -> Math Function/1
  w 1/1 -> vgw/1
  Sum2/1 -> 2.2/1
  12/1 -> Sum/4
  vgw_p2/1 -> w/2, 2.4/1
  2.4/1 -> Sum2/2
  w/1 -> 1/1, vgw_p3/1
  vgw_p3/1 -> 2/1, 2.1/1
  1/1 -> Sum/3
  2.1/1 -> Sum2/3
  " w"/1 -> Sum/2
  2/1 -> " w"/1
  2.2/1 -> w 1/2

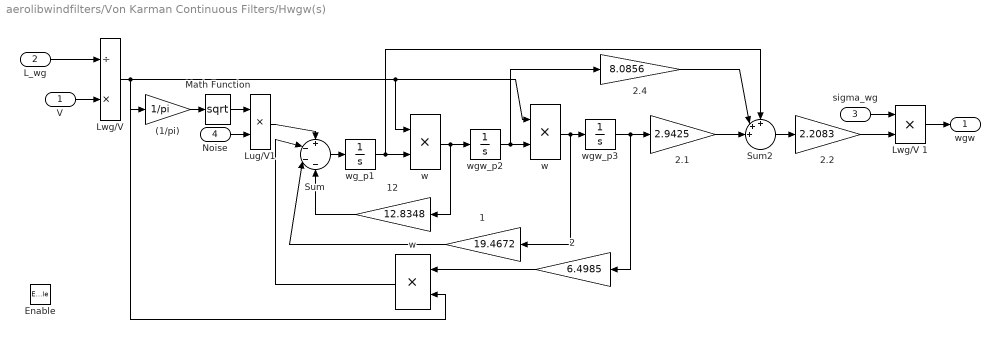
== system aerolibwindfilters/Von Karman Continuous Filters/Hwgw(s) ==
  V : Inport  LatchInput=off
  L_wg : Inport  Port=2  LatchInput=off
  sigma_wg : Inport  Port=3  LatchInput=off
  Noise : Inport  Port=4  LatchInput=off
  Enable : EnablePort  StatesWhenEnabling=reset
  " w" : Product  Orientation=left  SaturateOnIntegerOverflow=on  InputSameDT=on
  (1/pi) : Gain  Gain=1/pi  SaturateOnIntegerOverflow=on
  1 : Gain  Orientation=left  Gain=19.4672  SaturateOnIntegerOverflow=on
  12 : Gain  Orientation=left  Gain=12.8348  SaturateOnIntegerOverflow=on
  2 : Gain  Orientation=left  Gain=6.4985  SaturateOnIntegerOverflow=on
  2.1 : Gain  Gain=2.9425  SaturateOnIntegerOverflow=on
  2.2 : Gain  Gain=2.2083  SaturateOnIntegerOverflow=on
  2.4 : Gain  Gain=8.0856  SaturateOnIntegerOverflow=on
  Lug/V1 : Product  SaturateOnIntegerOverflow=on  InputSameDT=on
  Lwg/V : Product  Inputs=/*  SaturateOnIntegerOverflow=on  InputSameDT=on
  Lwg/V 1 : Product  SaturateOnIntegerOverflow=on  InputSameDT=on
  Math Function : Math  Operator=sqrt  SaturateOnIntegerOverflow=on
  Sum : Sum  Inputs=+---  SaturateOnIntegerOverflow=on  InputSameDT=on
  Sum2 : Sum  Inputs=+++||  SaturateOnIntegerOverflow=on  InputSameDT=on
  w : Product  SaturateOnIntegerOverflow=on  InputSameDT=on
  "w " : Product  SaturateOnIntegerOverflow=on  InputSameDT=on
  wg_p1 : Integrator
  wgw_p2 : Integrator
  wgw_p3 : Integrator
  wgw : Outport  OutputWhenDisabled=reset  InitialOutput=0
  wires:
  sigma_wg/1 -> Lwg/V 1/1
  Lwg/V 1/1 -> wgw/1
  Sum2/1 -> 2.2/1
  L_wg/1 -> Lwg/V/1
  V/1 -> Lwg/V/2
  Lwg/V/1 -> "w "/1, w/1, (1/pi)/1, " w"/2
  Math Function/1 -> Lug/V1/1
  Noise/1 -> Lug/V1/2
  Sum/1 -> wg_p1/1
  Lug/V1/1 -> Sum/1
  wg_p1/1 -> "w "/2, Sum2/1
  "w "/1 -> 12/1, wgw_p2/1
  (1/pi)/1 -> Math Function/1
  12/1 -> Sum/4
  wgw_p2/1 -> w/2, 2.4/1
  2.4/1 -> Sum2/2
  w/1 -> 1/1, wgw_p3/1
  wgw_p3/1 -> 2/1, 2.1/1
  1/1 -> Sum/3
  2.1/1 -> Sum2/3
  " w"/1 -> Sum/2
  2/1 -> " w"/1
  2.2/1 -> Lwg/V 1/2
